simulink model "sortie_photorecepteurs"  (R2021a)
settings: Solver=ode2  StartTime=0.0  StopTime=10.0  FixedStep=0.01  RelTol=1e-3
values from neighbouring files (symbols this model uses):
  A = matrice()    [Initialisation.m]    (also in matrice.m = zeros(taille_A))
  deltarho = 3.8    [matrice.m]    (also in sorties_photo.m)
  MurComplet = env()    [Initialisation.m]
  y = 500    [Initialisation.m]
undefined symbols (not defined in the file or in its folder): U, Y
libraries: simulink x1
settings Model: Creator=vincent  LastModifiedBy=Romain

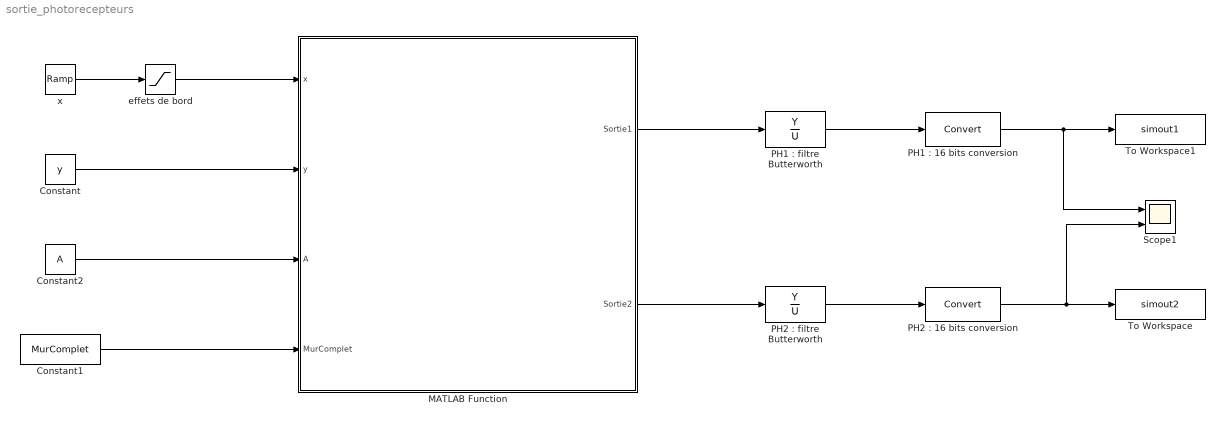
== system sortie_photorecepteurs ==
  Constant : Constant  Value=y
  Constant1 : Constant  Value=MurComplet
  Constant2 : Constant  Value=A
  MATLAB Function : MATLAB Function  Description=Contient le script sorties_photorecepteurs  TreatAsAtomicUnit=on
  "PH1 : 16 bits conversion" : DataTypeConversion  OutMax=[-1+2^16]
  "PH1 : filtre Butterworth" : DiscreteTransferFcn  Numerator=Y  Denominator=U
  "PH2 : 16 bits conversion" : DataTypeConversion  OutMax=[-1+2^16]
  "PH2 : filtre Butterworth" : DiscreteTransferFcn  Numerator=Y  Denominator=U
  Scope1 : Scope  NumInputPorts=2
  To Workspace : ToWorkspace  VariableName=simout2  SaveFormat=Timeseries  SampleTime=-1
  To Workspace1 : ToWorkspace  VariableName=simout1  SaveFormat=Timeseries  SampleTime=-1
  effets de bord : Saturate  UpperLimit=4000 - y*tan(deltarho/2)  LowerLimit=1 + y*tan(deltarho/2)
  x : simulink/Sources/Ramp  slope=500  start=0  InitialOutput=0
  wires:
  x/1 -> effets de bord/1
  "PH2 : filtre Butterworth"/1 -> "PH2 : 16 bits conversion"/1
  "PH1 : filtre Butterworth"/1 -> "PH1 : 16 bits conversion"/1
  MATLAB Function/2(Sortie2) -> "PH2 : filtre Butterworth"/1
  effets de bord/1 -> MATLAB Function/1(x)
  Constant/1 -> MATLAB Function/2(y)
  Constant2/1 -> MATLAB Function/3(A)
  Constant1/1 -> MATLAB Function/4(MurComplet)
  MATLAB Function/1(Sortie1) -> "PH1 : filtre Butterworth"/1
  "PH1 : 16 bits conversion"/1 -> Scope1/1, To Workspace1/1
  "PH2 : 16 bits conversion"/1 -> Scope1/2, To Workspace/1

== matlab function sortie_photorecepteurs/MATLAB Function ==
  data: x input; y input; A input; Sortie1 output size=1; Sortie2 output; MurComplet input
function [Sortie1,Sortie2] = sorties_photorecepteurs(x,y,A,MurComplet)
%-------------------------------------------------------------------------
%Constantes utiles
deltarho = (3.8*pi)/180 ; % largeur à mi-hauteur de la gaussienne
deltaphi = (3.8*pi)/180; % Angle inter-récepteur
step = 0.005; % Résolution de la matrice A

%-------------------------------------------------------------------------
% Recherche de Theta_n: l’ensemble de bords contrastés du Mur
i = 1;
j = 1;
Theta_n = zeros(1,400); % 400 = max transistions possibles
Indice_B_C = zeros(1,400);
while i < 4000 % On parcourt l'ensemble des valeurs du Mur
    teinte = MurComplet(i);
    while MurComplet(i) == teinte
        i = i+1;
        if i > 3999
            break
        end
    end % i correspond à une transition, on calcule donc l'angle correspondant
    Theta_n(j) = atan2(-y,i-x)*180/pi;
    % On sauvegarde les indices des bords contrastés du Mur
    Indice_B_C(j)=i; 
    j = j+1;
end
%-------------------------------------------------------------------------
%Sélection des angles de transistion dans le champs visuel du
%photorecepteur 1 et du photorecepteur 2
IndiceTheta1=Indice_B_C( (- 1.3*deltarho + deltaphi/2 - pi/2 <= Theta_n) & (Theta_n <= + 1.3*deltarho + deltaphi/2 - pi/2) );
IndiceTheta2=Indice_B_C((- 1.3*deltarho - deltaphi/2 - pi/2<= Theta_n) & (Theta_n <= + 1.3*deltarho - deltaphi/2 - pi/2) );

% Sauvegarde des valeurs correspondant aux angles précedents
Theta1 = Theta_n(IndiceTheta1);
Theta2 = Theta_n(IndiceTheta2);

% On "transforme" directement ces angles pour les utiliser comme indice
Theta1 = floor(abs(Theta1/step));
Theta2 = floor(abs(Theta2/step));

% Constantes utiles pour les conditions
tailleT1 = length(Theta1);
tailleT2 = length(Theta2);

%-------------------------------------------------------------------------
%Calcul des différentes sorties

Sortie1 = [0]; % Simulink n'accepte pas si Sortie1 est une constante
if(tailleT1 == 0) % Si aucune nuance de teinte n'est detectée
    indice = min(4000,floor(x+y*tan(deltaphi/2)));
    Sortie1(1) = MurComplet(indice); % On prend la teinte en face de l'oeil
elseif tailleT1 ==1
    % Une seule nuance de teinte detectée, on calcule la sortie à partir de
    % la teinte précedente et la teinte suivante
    Sortie1(1) = MurComplet(IndiceTheta1-1)*A(Theta1,1) + MurComplet(IndiceTheta1)*A(end,Theta2);
else % Plus d'une nuance de teinte detectée
    % On calcule chaque sortie d'après la formule
    Sortie1(1) = MurComplet(IndiceTheta1(1))*A(Theta1(1),1) + MurComplet(IndiceTheta1(end))*A(end,Theta1(end));
    for i= 2:(tailleT1-1)
        Sortie1(1) = Sortie1(1) + MurComplet(IndiceTheta1(i))*A(Theta1(i+1),Theta1(i));
    end
end    

Sortie2 = [0];% Simulink n'accepte pas si Sortie1 est une constante
if(tailleT2 == 0) % Si aucune nuance de teinte n'est detectée
    indice = min(4000,floor(x+y*tan(deltaphi/2)));
    Sortie2(1) = MurComplet(indice); % On prend la teinte en face de l'oeil
elseif tailleT2 ==1
    % Une seule nuance de teinte detectée, on calcule la sortie à partir de
    % la teinte précedente et la teinte suivante
    Sortie2(1) = MurComplet(IndiceTheta2-1)*A(Theta2,1) + MurComplet(IndiceTheta2)*A(end,Theta2);
else % Plus d'une nuance de teinte detectée
    % On calcule chaque sortie d'après la formule
    Sortie2(1) = MurComplet(IndiceTheta2(1))*A(Theta2(1),1) + MurComplet(IndiceTheta2(end))*A(end,Theta2(end));
    for i= 2:(tailleT2-1)
        Sortie2(1) = Sortie2(1) + MurComplet(IndiceTheta2(i))*A(Theta2(i+1),Theta2(i));
    end
end
